simulink model "hall_sensor"  (R2023a)
settings: configuration reference "config" (kept outside this file)
model workspace (MAT data in the model file):
  x = Simulink.Signal
  x.Description = 'x 状态变量'
  x.DataType = 'single'
  x.Dimensions = -1
  x.DimensionsMode = 'auto'
  x.Complexity = 'auto'
  x.SampleTime = -1
  x.SamplingMode = 'auto'
  x.InitialValue = '0'
settings Model: DataDictionary=model_config.sldd  Creator=huangcheng  LastModifiedBy=Administrator
settings ConfigSetRef: SourceName=config

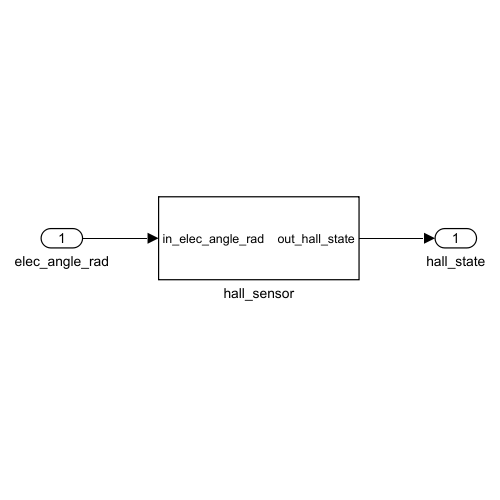
[thumbnail: Simulink's stored preview of the top-level diagram]
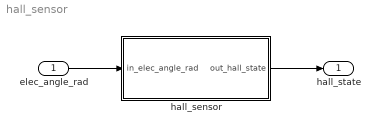
== system hall_sensor ==
  elec_angle_rad : Inport  OutDataTypeStr=single
  hall_sensor : Subsystem
  hall_state : Outport  OutDataTypeStr=uint8
  wires:
  elec_angle_rad/1 -> hall_sensor/1(in_elec_angle_rad)
  hall_sensor/1(out_hall_state) -> hall_state/1

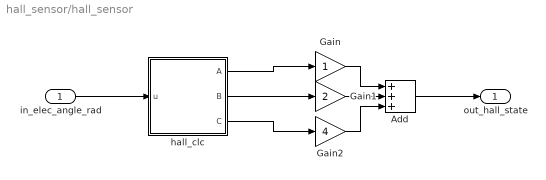
== system hall_sensor/hall_sensor ==
  in_elec_angle_rad : Inport  OutDataTypeStr=single
  Add : Sum  Inputs=+++
  Gain : Gain  OutDataTypeStr=uint8
  Gain1 : Gain  Gain=2  OutDataTypeStr=uint8
  Gain2 : Gain  Gain=4  OutDataTypeStr=uint8
  hall_clc : MATLAB Function  TreatAsAtomicUnit=on
  out_hall_state : Outport  OutDataTypeStr=uint8
  wires:
  hall_clc/3(C) -> Gain2/1
  Add/1 -> out_hall_state/1
  hall_clc/1(A) -> Gain/1
  Gain1/1 -> Add/2
  Gain/1 -> Add/1
  in_elec_angle_rad/1 -> hall_clc/1(u)
  hall_clc/2(B) -> Gain1/1
  Gain2/1 -> Add/3

== matlab function hall_sensor/hall_clc ==
  data: u input; A output; B output; C output
function [A,B,C] = HALL_Sensro(u)
sita = u*360/(2*pi);

if (sita>=0 && sita<30) || (sita>=330 && sita<=360)
    A = 1;
    B = 1;
    C = 0;
elseif sita>=30 && sita<90
    A = 0;
    B = 1;
    C = 0;
elseif sita >=90 && sita <150
    A = 0;
    B = 1;
    C = 1;
elseif sita >=150 && sita <210
    A = 0;
    B = 0;
    C = 1;
elseif sita >=210 && sita <270
    A = 1;
    B = 0;
    C = 1;
elseif sita >=270 && sita <330
    A = 1;
    B = 0;
    C = 0;
else 
    A = 0;
    B = 0;
    C = 0;
end
